simulink model "task4simulinkmodel"  (R2025b)
settings: Solver=VariableStepAuto  StartTime=0.0  StopTime=90  RelTol=1e-3
values from neighbouring files (symbols this model uses):
  C1 = 700    [Task_1.m]    (also in task_4.m)
  C2 = C2_sport    (= 1500)    [Task_1.m]    (also in task_4.m)
  C3 = 300    [Task_1.m]    (also in task_4.m)
  K1 = 2200    [Task_1.m]    (also in task_4.m)
  K2 = K2_sport    (= 13000)    [Task_1.m]    (also in task_4.m)
  K3 = 120000    [Task_1.m]    (also in task_4.m)
  M1 = 50    [Task_1.m]    (also in task_4.m)
  M2 = 250    [Task_1.m]    (also in task_4.m)
  M3 = 100    [Task_1.m]    (also in task_4.m)
settings Model: Creator=co1il  LastModifiedBy=ugoor
settings SolverCC: AlgebraicLoopSolver=TrustRegion
settings DataIOCC: ReturnWorkspaceOutputs=off
settings DebuggingCC: UnconnectedInputMsg=warning  UnconnectedOutputMsg=warning  UnconnectedLineMsg=warning  PregeneratedLibrarySubsystemCodeDiagnostic=none  ArithmeticOperatorsInVariantConditions=warning
settings ModelReferenceCC: EnableRefExpFcnMdlSchedulingChecks=on
settings SFSimCC: SimUseLocalCustomCode=off  CustomCodeUndefinedFunction=UseInterfaceOnly
settings RTWCC: RTWUseLocalCustomCode=off  GPUComputeCapability=3.5
settings CodeAppCC: StateflowObjectComments=on

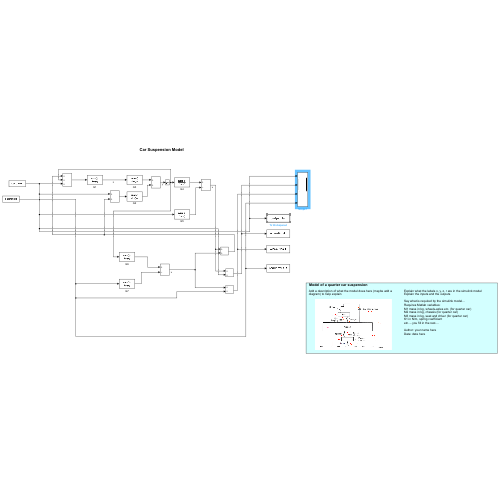
[thumbnail: Simulink's stored preview of the top-level diagram]
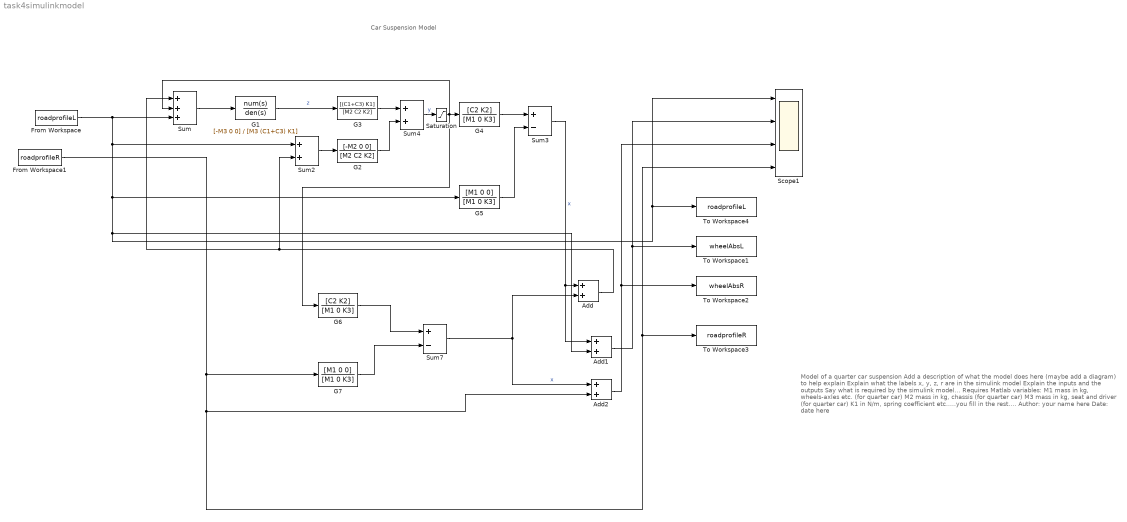
== system task4simulinkmodel ==
  note: Model of a quarter car suspension
      |
      | Add a description of what the model does here (maybe add a diagram) to help explain
      |
      | Explain what the labels x, y, z, r are in the simulink model
      | Explain the inputs and the outputs
      |
      | Say what is required by the simulink model...
      | Requires Matlab variables:
      | M1 mass in kg, wheels-axles etc. (for quarter car)
      | M2 mass in kg, chassis (for quarter car)
      | M3 mass in kg, seat and driver (for quarter car)
      | K1 in N/m, spring coefficient
      | etc.....you fill in the rest....
      |
      | Author: your name here
      | Date: date here
  note: Car Suspension Model
  Add : Sum
  Add1 : Sum
  Add2 : Sum
  From Workspace : FromWorkspace  VariableName=roadprofileL  SampleTime=1
  From Workspace1 : FromWorkspace  VariableName=roadprofileR  SampleTime=1
  G1 : TransferFcn  Numerator=[-M3 0 0]  Denominator=[M3 (C1+C3) K1]
  G2 : TransferFcn  Numerator=[-M2 0 0]  Denominator=[M2 C2 K2]
  G3 : TransferFcn  Numerator=[(C1+C3) K1]  Denominator=[M2 C2 K2]
  G4 : TransferFcn  Numerator=[C2 K2]  Denominator=[M1 0 K3]
  G5 : TransferFcn  Numerator=[M1 0 0]  Denominator=[M1 0 K3]
  G6 : TransferFcn  Numerator=[C2 K2]  Denominator=[M1 0 K3]
  G7 : TransferFcn  Numerator=[M1 0 0]  Denominator=[M1 0 K3]
  Saturation : Saturate  UpperLimit=0.02  LowerLimit=-0.02  LinearizeAsGain=off
  Scope1 : Scope  NumInputPorts=4
      settings: ActiveDisplayYMinimum=-0.045032224133995886  ActiveDisplayYMaximum=0.038645182526129043
  Sum : Sum  Inputs=+++
  Sum2 : Sum
  Sum3 : Sum  Inputs=+-
  Sum4 : Sum
  Sum7 : Sum  Inputs=+-
  To Workspace1 : ToWorkspace  VariableName=wheelAbsL  SaveFormat=Timeseries  SampleTime=1
  To Workspace2 : ToWorkspace  VariableName=wheelAbsR  SaveFormat=Timeseries  SampleTime=1
  To Workspace3 : ToWorkspace  VariableName=roadprofileR  SaveFormat=Timeseries  SampleTime=1
  To Workspace4 : ToWorkspace  VariableName=roadprofileL  SaveFormat=Timeseries  SampleTime=1
  wires:
  G1/1 -> G3/1  "z"
  Sum/1 -> G1/1
  Sum2/1 -> G2/1
  G4/1 -> Sum3/1
  G5/1 -> Sum3/2
  G2/1 -> Sum4/2
  G3/1 -> Sum4/1
  From Workspace/1 -> Sum2/1, To Workspace4/1, Scope1/1, Add1/2, G5/1, Sum/3
  Sum4/1 -> Saturation/1  "y"
  Saturation/1 -> G6/1, Sum/2, G4/1
  G6/1 -> Sum7/1
  G7/1 -> Sum7/2
  From Workspace1/1 -> Scope1/4, To Workspace3/1, Add2/2, G7/1
  Sum3/1 -> Add1/1, Add/1  "x"
  Sum7/1 -> Add/2, Add2/1  "x"
  Add/1 -> Sum/1, Sum2/2
  Add1/1 -> To Workspace1/1, Scope1/2
  Add2/1 -> To Workspace2/1, Scope1/3
